simulink model "dron_thrust_pos"  (R2022b)
settings: Solver=VariableStepAuto  StartTime=0.0  StopTime=8  RelTol=1e-3
values from neighbouring files (symbols this model uses):
  air_density = 1.225    [matlab.mat]
  drag_coef = 1    [matlab.mat]
  front_area = 0.02    [matlab.mat]
  g = 9.8    [matlab.mat]
  I_x = 0.0042    [matlab.mat]
  I_y = 0.0042    [matlab.mat]
  I_z = 0.0125    [matlab.mat]
  motor_force = 2    [matlab.mat]
  motor_metrix = [1 1 1 1 0.97 0.97 1 1 1 1 1 1 ... (36 elements, 4x9)]    [matlab.mat]
  motor_thrust_coeff = 4.5e-06    [matlab.mat]
  motor_torque_coeff = 9.0957049977e-08    [matlab.mat]
  side_rode_len = 0.0707106781187    [matlab.mat]
  total_mass = 0.4    [matlab.mat]
libraries: simulink x4, uavutilslib x1
settings Model: Creator=NIRMIT  LastModifiedBy=NIRMIT

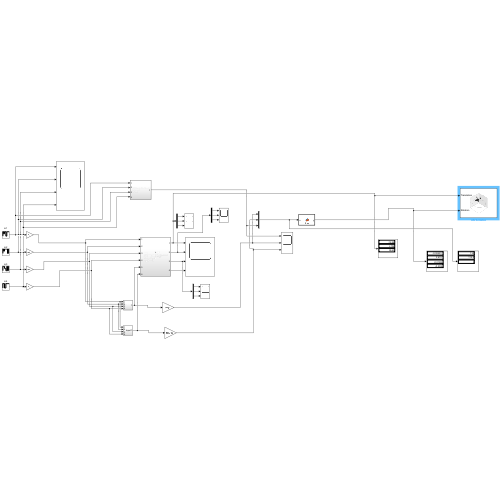
[thumbnail: Simulink's stored preview of the top-level diagram]
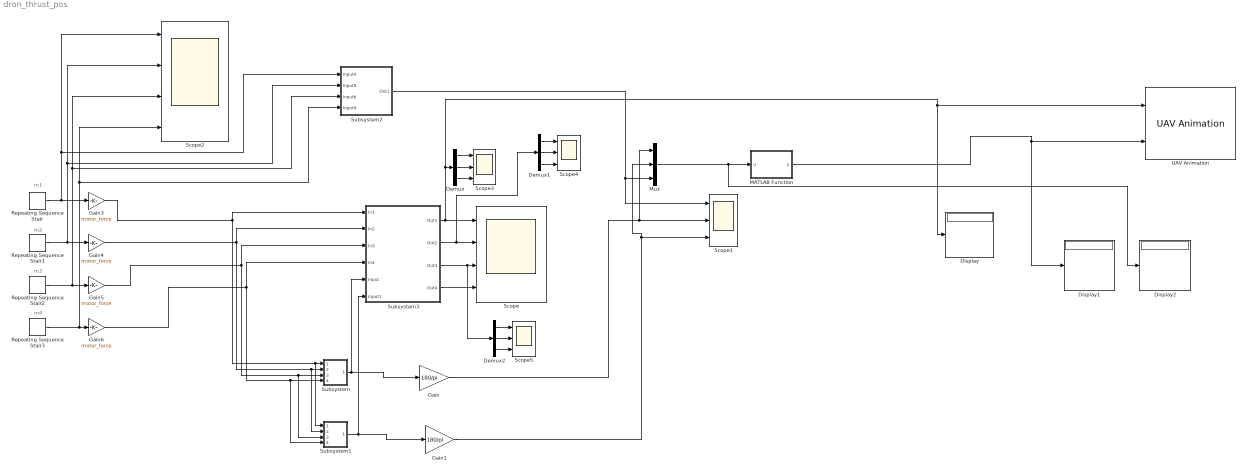
== system dron_thrust_pos ==
  note: m4
  note: m3
  note: m2
  note: m1
  Demux : Demux  Outputs=3
  Demux1 : Demux  Outputs=3
  Demux2 : Demux  Outputs=3
  Display : Display
  Display1 : Display
  Display2 : Display
  Gain : Gain  Gain=180/pi
  Gain1 : Gain  Gain=180/pi
  Gain{3..6} (4 alike) : Gain  Gain=motor_force
  MATLAB Function : MATLAB Function  TreatAsAtomicUnit=on
  Mux : Mux  Inputs=3
  Repeating Sequence Stair : simulink/Sources/Repeating Sequence Stair  OutValues=motor_metrix(1,:)  tsamp=1  OutMin=[]  OutMax=[]  OutDataTypeStr=double  OutputDataTypeScalingMode=double  OutDataType=fixdt(0,8)  ConRadixGroup=Best Precision: Vector-wise  OutScaling=2^-12
  Repeating Sequence Stair1 : simulink/Sources/Repeating Sequence Stair  OutValues=motor_metrix(2,:)  tsamp=1  OutMin=[]  OutMax=[]  OutDataTypeStr=double  OutputDataTypeScalingMode=double  OutDataType=fixdt(0,8)  ConRadixGroup=Best Precision: Vector-wise  OutScaling=2^-12
  Repeating Sequence Stair2 : simulink/Sources/Repeating Sequence Stair  OutValues=motor_metrix(3,:)  tsamp=1  OutMin=[]  OutMax=[]  OutDataTypeStr=double  OutputDataTypeScalingMode=double  OutDataType=fixdt(0,8)  ConRadixGroup=Best Precision: Vector-wise  OutScaling=2^-12
  Repeating Sequence Stair3 : simulink/Sources/Repeating Sequence Stair  OutValues=motor_metrix(4,:)  tsamp=1  OutMin=[]  OutMax=[]  OutDataTypeStr=double  OutputDataTypeScalingMode=double  OutDataType=fixdt(0,8)  ConRadixGroup=Best Precision: Vector-wise  OutScaling=2^-12
  Scope : Scope  NumInputPorts=4
  Scope{1,3..5} (4 alike) : Scope  NumInputPorts=3
  Scope2 : Scope  NumInputPorts=4
  Subsystem : Subsystem
  Subsystem1 : Subsystem
  Subsystem2 : Subsystem
  Subsystem3 : Subsystem
  UAV Animation : uavutilslib/UAV Animation  UAVType=Multirotor  UAVSize=1  InertialZDirection=Up  SampleTime=-1
  wires:
  Gain3/1 -> Subsystem1/1(In1), Subsystem/1(Input), Subsystem3/1(In1)
  Gain4/1 -> Subsystem3/2(In2), Subsystem1/2(In3), Subsystem/2(Input1)
  Gain5/1 -> Subsystem3/3(In3), Subsystem/3(Input2), Subsystem1/3(In4)
  Gain6/1 -> Subsystem3/4(In4), Subsystem/4(Input3), Subsystem1/4(In2)
  Subsystem2/1(Out1) -> Mux/3, Scope1/1
  Subsystem/1(Out1) -> Gain/1, Subsystem3/5(Input)
  Subsystem1/1(Input1) -> Subsystem3/6(Input1), Gain1/1
  Repeating Sequence Stair3/1 -> Scope2/4, Subsystem2/4(Input9), Gain6/1
  Repeating Sequence Stair2/1 -> Gain5/1, Scope2/3, Subsystem2/3(Input6)
  Repeating Sequence Stair1/1 -> Gain4/1, Scope2/2, Subsystem2/2(Input8)
  Repeating Sequence Stair/1 -> Gain3/1, Scope2/1, Subsystem2/1(Input4)
  Subsystem3/2(Out2) -> Demux1/1, Scope/2
  Subsystem3/3(Out3) -> Demux2/1, Scope/3
  Subsystem3/4(Out4) -> Scope/4
  Gain/1 -> Mux/1, Scope1/2
  Gain1/1 -> Mux/2, Scope1/3
  Demux/2 -> Scope3/2
  Demux/1 -> Scope3/1
  Demux/3 -> Scope3/3
  Demux1/1 -> Scope4/1
  Demux1/2 -> Scope4/2
  Demux1/3 -> Scope4/3
  Demux2/1 -> Scope5/1
  Demux2/2 -> Scope5/2
  Demux2/3 -> Scope5/3
  Mux/1 -> Display2/1, MATLAB Function/1(u)
  MATLAB Function/1(y) -> Display1/1, UAV Animation/2
  Subsystem3/1(Out1) -> UAV Animation/1, Display/1, Demux/1, Scope/1

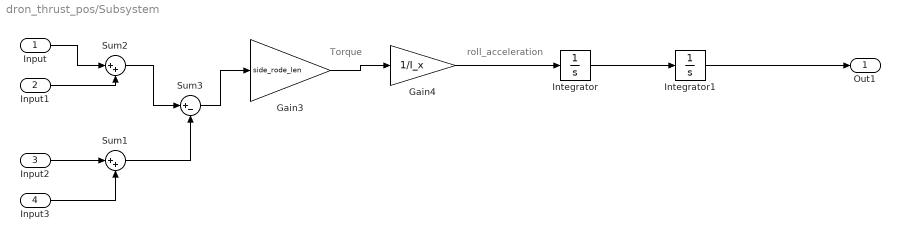
== system dron_thrust_pos/Subsystem ==
  note: roll_acceleration
  note: Torque
  Input : Inport
  Input1 : Inport  Port=2
  Input2 : Inport  Port=3
  Input3 : Inport  Port=4
  Gain3 : Gain  Gain=side_rode_len
  Gain4 : Gain  Gain=1/I_x
  Integrator : Integrator
  Integrator1 : Integrator
  Sum1 : Sum  Inputs=|++
  Sum2 : Sum  Inputs=|++
  Sum3 : Sum  Inputs=|+-
  Out1 : Outport
  wires:
  Input1/1 -> Sum2/2
  Input/1 -> Sum2/1
  Gain3/1 -> Gain4/1
  Input2/1 -> Sum1/1
  Input3/1 -> Sum1/2
  Sum1/1 -> Sum3/2
  Sum2/1 -> Sum3/1
  Sum3/1 -> Gain3/1
  Gain4/1 -> Integrator/1
  Integrator/1 -> Integrator1/1
  Integrator1/1 -> Out1/1

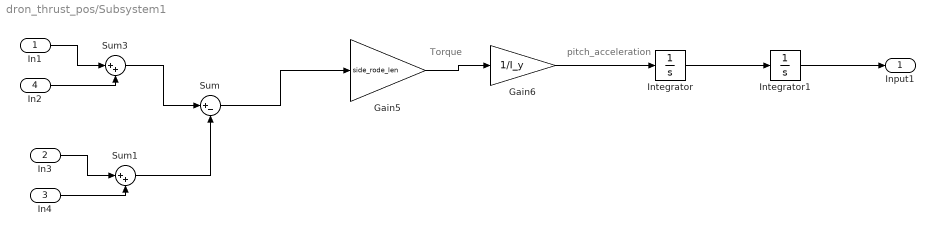
== system dron_thrust_pos/Subsystem1 ==
  note: Torque
  note: pitch_acceleration
  In1 : Inport
  In3 : Inport  Port=2
  In4 : Inport  Port=3
  In2 : Inport  Port=4
  Gain5 : Gain  Gain=side_rode_len
  Gain6 : Gain  Gain=1/I_y
  Integrator : Integrator
  Integrator1 : Integrator
  Sum : Sum  Inputs=|+-
  Sum1 : Sum  Inputs=|++
  Sum3 : Sum  Inputs=|++
  Input1 : Outport
  wires:
  Gain5/1 -> Gain6/1
  In2/1 -> Sum3/2
  In1/1 -> Sum3/1
  In3/1 -> Sum1/1
  In4/1 -> Sum1/2
  Sum1/1 -> Sum/2
  Sum3/1 -> Sum/1
  Sum/1 -> Gain5/1
  Gain6/1 -> Integrator/1
  Integrator/1 -> Integrator1/1
  Integrator1/1 -> Input1/1

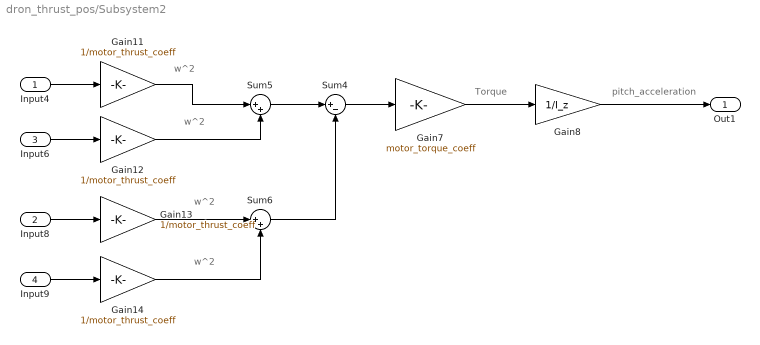
== system dron_thrust_pos/Subsystem2 ==
  note: w^2
  note: Torque
  note: pitch_acceleration
  note: w^2
  note: w^2
  note: w^2
  Input4 : Inport
  Input8 : Inport  Port=2
  Input6 : Inport  Port=3
  Input9 : Inport  Port=4
  Gain{11..14} (4 alike) : Gain  Gain=1/motor_thrust_coeff
  Gain7 : Gain  Gain=motor_torque_coeff
  Gain8 : Gain  Gain=1/I_z
  Sum4 : Sum  Inputs=|+-
  Sum5 : Sum  Inputs=|++
  Sum6 : Sum  Inputs=|++
  Out1 : Outport
  wires:
  Input6/1 -> Gain12/1
  Input8/1 -> Gain13/1
  Sum6/1 -> Sum4/2
  Sum4/1 -> Gain7/1
  Input9/1 -> Gain14/1
  Gain14/1 -> Sum6/2
  Gain11/1 -> Sum5/1
  Gain13/1 -> Sum6/1
  Sum5/1 -> Sum4/1
  Gain12/1 -> Sum5/2
  Gain7/1 -> Gain8/1
  Input4/1 -> Gain11/1
  Gain8/1 -> Out1/1

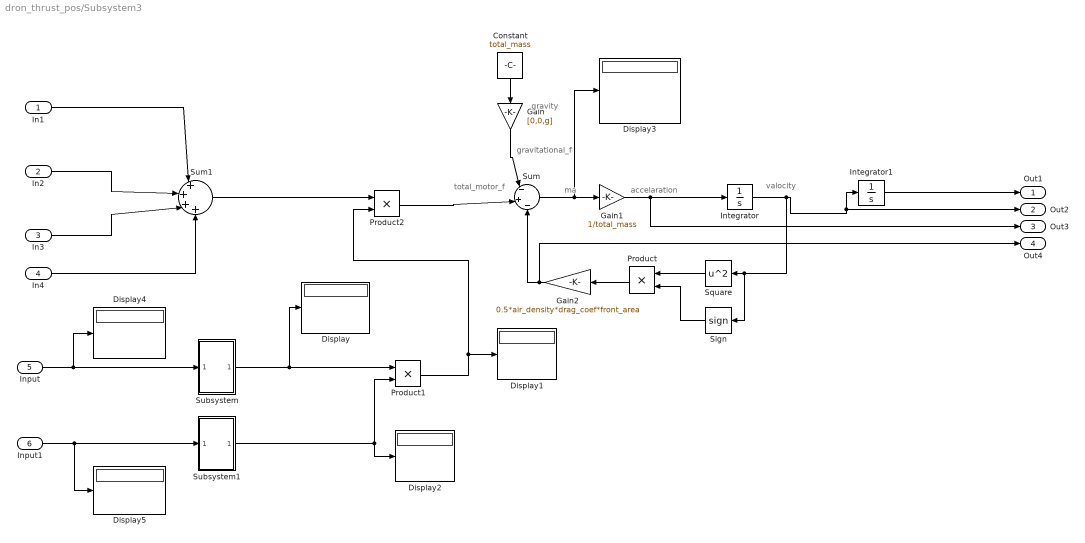
== system dron_thrust_pos/Subsystem3 ==
  note: valocity
  note: accelaration
  note: ma
  note: gravitational_f
  note: total_motor_f
  note: gravity
  In1 : Inport
  In2 : Inport  Port=2
  In3 : Inport  Port=3
  In4 : Inport  Port=4
  Input : Inport  Port=5
  Input1 : Inport  Port=6
  Constant : Constant  Value=total_mass
  Display{,1..5} (6 alike) : Display
  Gain : Gain  Gain=[0,0,g]
  Gain1 : Gain  Gain=1/total_mass
  Gain2 : Gain  Gain=0.5*air_density*drag_coef*front_area
  Integrator : Integrator
  Integrator1 : Integrator
  Product : Product
  Product1 : Product
  Product2 : Product
  Sign : Signum
  Square : Math  Operator=square
  Subsystem : Subsystem
  Subsystem1 : Subsystem
  Sum : Sum  Inputs=|-|+|-
  Sum1 : Sum  Inputs=|+|+|+|+
  Out1 : Outport
  Out2 : Outport  Port=2
  Out3 : Outport  Port=3
  Out4 : Outport  Port=4
  wires:
  Gain1/1 -> Out3/1, Integrator/1
  Gain2/1 -> Out4/1, Sum/3
  Sign/1 -> Product/2
  Sum/1 -> Display3/1, Gain1/1
  Constant/1 -> Gain/1
  In1/1 -> Sum1/1
  Gain/1 -> Sum/1
  Product/1 -> Gain2/1
  Integrator/1 -> Sign/1, Square/1, Out2/1, Integrator1/1
  Square/1 -> Product/1
  Integrator1/1 -> Out1/1
  In4/1 -> Sum1/4
  In3/1 -> Sum1/3
  In2/1 -> Sum1/2
  Input/1 -> Display4/1, Subsystem/1(In1)
  Subsystem/1(Out1) -> Display/1, Product1/1
  Input1/1 -> Display5/1, Subsystem1/1(In1)
  Subsystem1/1(Out1) -> Display2/1, Product1/2
  Product2/1 -> Sum/2
  Product1/1 -> Display1/1, Product2/2
  Sum1/1 -> Product2/1

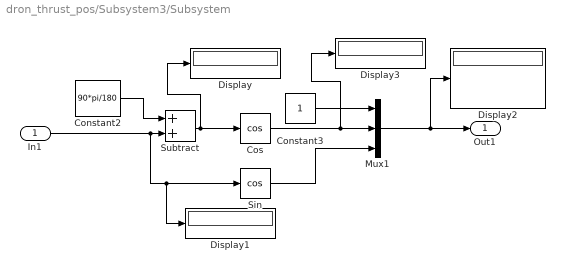
== system dron_thrust_pos/Subsystem3/Subsystem ==
  In1 : Inport
  Constant2 : Constant  Value=90*pi/180
  Constant3 : Constant
  Cos : Trigonometry  Operator=cos
  Display{,1..3} (4 alike) : Display
  Mux1 : Mux  Inputs=3
  Sin : Trigonometry  Operator=cos
  Subtract : Sum
  Out1 : Outport
  wires:
  Constant3/1 -> Mux1/1
  Constant2/1 -> Subtract/1
  Sin/1 -> Mux1/3
  Cos/1 -> Display3/1, Mux1/2
  Subtract/1 -> Display/1, Cos/1
  Mux1/1 -> Display2/1, Out1/1
  In1/1 -> Display1/1, Sin/1, Subtract/2

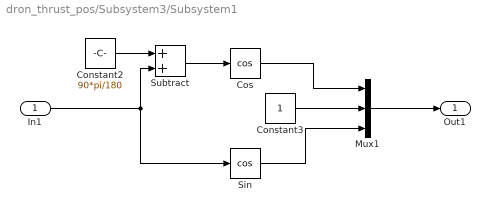
== system dron_thrust_pos/Subsystem3/Subsystem1 ==
  In1 : Inport
  Constant2 : Constant  Value=90*pi/180
  Constant3 : Constant
  Cos : Trigonometry  Operator=cos
  Mux1 : Mux  Inputs=3
  Sin : Trigonometry  Operator=cos
  Subtract : Sum
  Out1 : Outport
  wires:
  Cos/1 -> Mux1/1
  Sin/1 -> Mux1/3
  In1/1 -> Sin/1, Subtract/2
  Mux1/1 -> Out1/1
  Constant2/1 -> Subtract/1
  Subtract/1 -> Cos/1
  Constant3/1 -> Mux1/2

== matlab function dron_thrust_pos/MATLAB Function ==
  data: u input; y output
function y = fcn(u)
y = eul2quat(u');
end
